simulink model "CounterEnabledSubsystem"  (R2022b)
settings: Solver=VariableStepAuto  StartTime=0.0  StopTime=inf  RelTol=1e-3
settings Model: Creator=Mo_7atem  LastModifiedBy=Mo_7atem

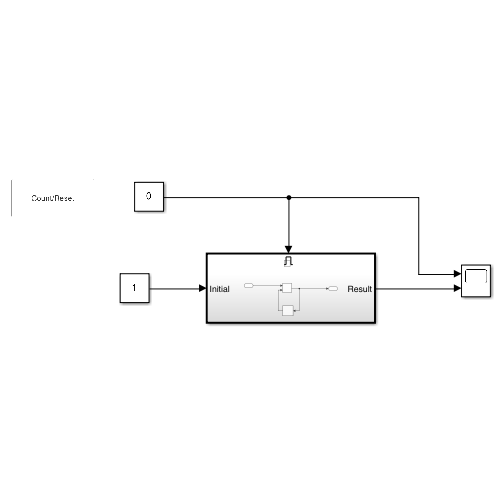
[thumbnail: Simulink's stored preview of the top-level diagram]
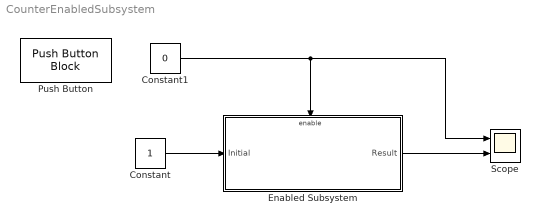
== system CounterEnabledSubsystem ==
  Constant : Constant
  Constant1 : Constant  Value=0
  Enabled Subsystem : Subsystem  TreatAsAtomicUnit=on
  Push Button : PushButtonBlock  ButtonText=Count/Reset  ButtonType=Latch  OffValue=0.000000
  Scope : Scope  NumInputPorts=2
  wires:
  Enabled Subsystem/1(Result) -> Scope/2
  Constant/1 -> Enabled Subsystem/1(Initial)
  Constant1/1 -> Scope/1, Enabled Subsystem/Enable

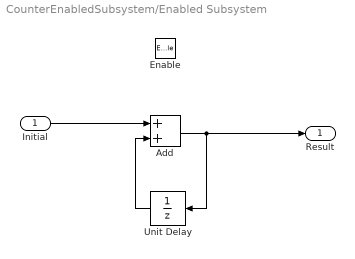
== system CounterEnabledSubsystem/Enabled Subsystem ==
  Initial : Inport
  Enable : EnablePort  StatesWhenEnabling=reset
  Add : Sum
  Unit Delay : UnitDelay  SampleTime=-1  HasFrameUpgradeWarning=on
  Result : Outport
  wires:
  Initial/1 -> Add/1
  Unit Delay/1 -> Add/2
  Add/1 -> Result/1, Unit Delay/1
